simulink model "YawRateController"  (R2024b)
settings: Solver=VariableStepAuto  StartTime=0.0  StopTime=10.0  RelTol=1e-3
libraries: slpidlib x1, vehdynlibscenariocommon x1, autolibshared x1
settings Model: Creator=aditya  LastModifiedBy=aditya

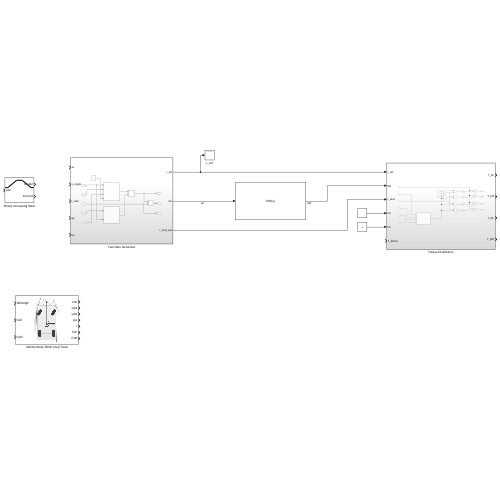
[thumbnail: Simulink's stored preview of the top-level diagram]
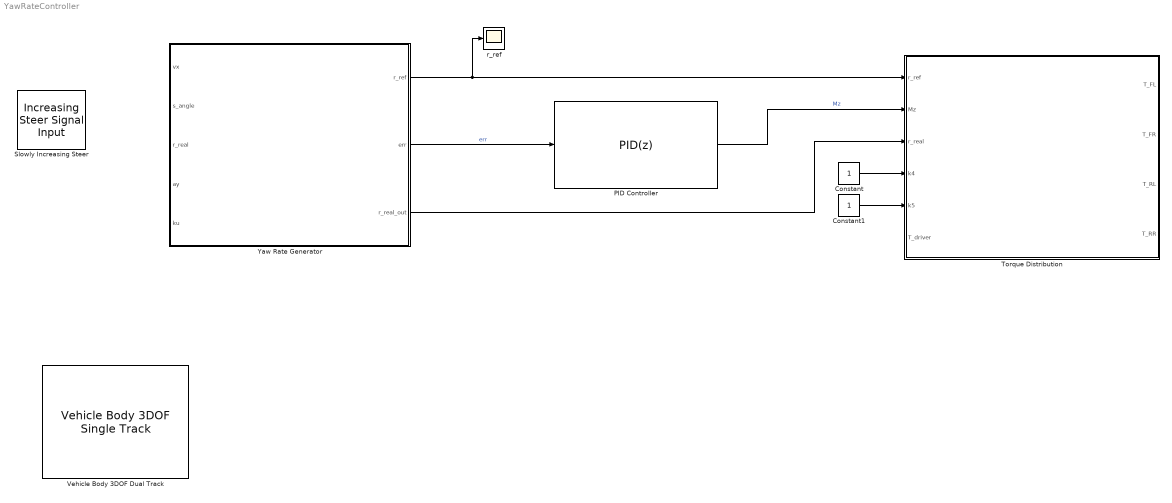
== system YawRateController ==
  Constant : Constant
  Constant1 : Constant
  PID Controller : slpidlib/PID Controller  Controller=PID  Form=Parallel  TimeDomain=Discrete-time  UseExternalTs=off  SampleTime=-1  IntegratorMethod=Forward Euler  FilterMethod=Forward Euler  ControllerParametersSource=internal  P=1  I=0  UseKiTs=off  D=0  UseExternalDerivativeSource=off  N=100  UseFilter=on  TunerSelectOption=Transfer Function Based (PID Tuner App)  InitialConditionSource=internal  InitialConditionForIntegrator=0  InitialConditionForFilter=0  DifferentiatorICPrevScaledInput=0  ExternalReset=none  TrackingMode=off  Kt=1  LimitOutput=off  SatLimitsSource=internal  UpperSaturationLimit=inf  LowerSaturationLimit=-inf  LinearizeAsGain=on  AntiWindupMode=none  Kb=1  LimitIntegrator=off  UpperIntegratorSaturationLimit=inf  LowerIntegratorSaturationLimit=-inf  POutMin=[]  POutMax=[]  IOutMin=[]  IOutMax=[]  DOutMin=[]  DOutMax=[]  NOutMin=[]  NOutMax=[]  SumOutMin=[]  SumOutMax=[]  SaturationOutMin=[]  SaturationOutMax=[]  PParamMin=[]  PParamMax=[]  IParamMin=[]  IParamMax=[]  DParamMin=[]  DParamMax=[]  NParamMin=[]  NParamMax=[]  KbParamMin=[]  KbParamMax=[]  KtParamMin=[]  KtParamMax=[]  KbOutMin=[]  KbOutMax=[]  KtOutMin=[]  KtOutMax=[]  IntegratorOutMin=[]  IntegratorOutMax=[]  FilterOutMin=[]  FilterOutMax=[]  SumI1OutMin=[]  SumI1OutMax=[]  SumI2OutMin=[]  SumI2OutMax=[]  SumI3OutMin=[]  SumI3OutMax=[]  SumI4OutMin=[]  SumI4OutMax=[]  SumDOutMin=[]  SumDOutMax=[]  DifferentiatorOutMin=[]  DifferentiatorOutMax=[]  FilterDiffOutCoefMin=[]  FilterDiffOutCoefMax=[]  ReciprocalOutMin=[]  ReciprocalOutMax=[]  SumDenOutMin=[]  SumDenOutMax=[]  SumNumOutMin=[]  SumNumOutMax=[]  DivideOutMin=[]  DivideOutMax=[]  UdiffTsProdOutMin=[]  UdiffTsProdOutMax=[]  NTsProdOutMin=[]  NTsProdOutMax=[]  UintegralTsProdOutMin=[]  UintegralTsProdOutMax=[]  UngainTsProdOutMin=[]  UngainTsProdOutMax=[]  ClampingZeroOutDataTypeStr=Inherit: Inherit via back propagation  ClampingZeroOutMin=[]  ClampingZeroOutMax=[]  FilterDenConstantOutDataTypeStr=Inherit: Inherit via back propagation  FilterDenConstantOutMin=[]  FilterDenConstantOutMax=[]  PCopyOutDataTypeStr=Inherit: Inherit via back propagation  PCopyOutMin=[]  PCopyOutMax=[]  NCopyOutDataTypeStr=Inherit: Inherit via back propagation  NCopyOutMin=[]  NCopyOutMax=[]  IntegratorContinuousStateAttributes=''  IntegratorStateMustResolveToSignalObject=off  IntegratorRTWStateStorageClass=Auto  FilterContinuousStateAttributes=''  FilterStateMustResolveToSignalObject=off  FilterRTWStateStorageClass=Auto  ParallelPVariant=InternalParameters  IdealPVariant=Disabled  IVariant=InternalParameters  DVariant=InternalParameters  IntegratorVariant=Discrete  SatVariant=Disabled  AWVariant=Passthrough  PCopyVariant=Disabled  TRVariant=Disabled  FdbkBlocksVariant=Forward  IdealPFdbkVariant=Disabled  SatFdbkVariant=Disabled  DerivativeFilterVariant=ForwardEulerFilter  NVariant=InternalParameters  NCopyVariant=Disabled  FilterICVariant=InternalICsFilter  IntegratorICVariant=InternalICs  ExternalResetVariant=Disabled  TRSumVariant=Passthrough  SumFdbkVariant=Disabled  SumVariant=Sum_PID  TsampFilterVariant=InternalTs  TsampNgainVariant=Passthrough  TsampIntegralVariant=Disabled_SignalSpec  ExternalSaturationOutDataTypeStr=Inherit: Same as second input  DerivativeSourceVariant=ErrorSignal  PreIntVariant=InternalPreInt
  Slowly Increasing Steer : vehdynlibscenariocommon/Increasing Steer Signal Input  ssMode=Initialize from model  ssVar=is50mph  tStart=2  velRef=50  velRefUnit=mph  steerRate=10  steerAmp=100  tDwellSteer=0  ayMax=.5  steerDir=Right  ayStop=off  ssDefault=on  X_o=0  Y_o=0  psi_o=0  ssTol=.1  ssMaxTime=30  ssWSName=is50mph  aMode=2
      settings: LibrarySourceBlock=vehdynlibscenario/Slowly Increasing Steer
  Torque Distribution : Subsystem
  Vehicle Body 3DOF Dual Track : autolibshared/Vehicle Body 3DOF Single Track  trackMode=Dual  inputMode=External forces  frontSteerMode=on  rearSteerMode=off  windMode=off  muMode=off  extFMode=off  extMMode=off  htchFMode=off  htchMMode=off  extXo=off  extpsio=off  extxdoto=off  extro=off  extYo=off  extTamb=off  extydoto=off  aMode=2  NF=2  NR=2  m=295  a=0.85  b=0.7  h=0.4  dh=1  hh=0.2  X_o=0  xdot_o=0  CalphaMode=off  sigmaMode=on  d=0  hl=0  w=[1.1,1.1]  Cy_f=12e3  Cy_r=11e3  sigma_f=.1  sigma_r=.1  alpha_f_brk=[-.1 .1]  Cy_f_data=[-9e3 9e3]  alpha_r_brk=[-.1 .1]  Cy_r_data=[-9e3 9e3]  Y_o=0  ydot_o=0  Izz=4000  psi_o=0  r_o=0  Af=0.728  Cd=0.85  Cl=.1  Cpm=.1  beta_w=[0 0.01:0.01:0.3]  Cs=[0:0.03:0.9]  Cym=[0 1e-6:0.01:0.3]  Pabs=101325  Tair=273  g=9.81  mu=1  xdot_tol=.01  Fznom=5000  Fxtire_sat=7e4  Fytire_sat=7e4  longOff=0  latOff=0  vertOff=0  wrapAng=off
      settings: LibrarySourceBlock=vehdynlibeom/Vehicle Body 3DOF Dual Track
  Yaw Rate Generator : Subsystem
  r_ref : Scope
  wires:
  Yaw Rate Generator/2(err) -> PID Controller/1  "err"
  PID Controller/1 -> Torque Distribution/2(Mz)  "Mz"
  Yaw Rate Generator/3(r_real_out) -> Torque Distribution/3(r_real)
  Yaw Rate Generator/1(r_ref) -> r_ref/1, Torque Distribution/1(r_ref)
  Constant/1 -> Torque Distribution/4(k4)
  Constant1/1 -> Torque Distribution/5(k5)

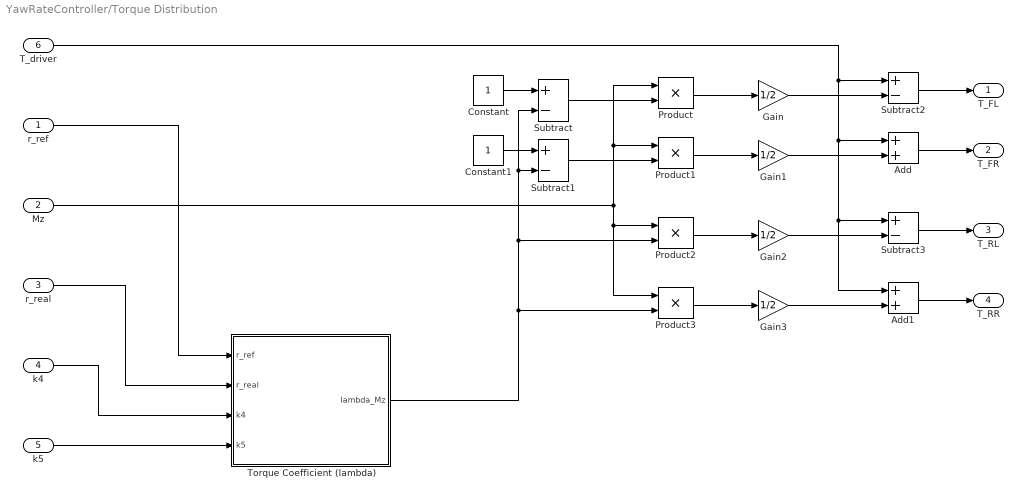
== system YawRateController/Torque Distribution ==
  r_ref : Inport
  Mz : Inport  Port=2
  r_real : Inport  Port=3
  k4 : Inport  Port=4
  k5 : Inport  Port=5
  T_driver : Inport  Port=6
  Add : Sum
  Add1 : Sum
  Constant : Constant
  Constant1 : Constant
  Gain{,1..3} (4 alike) : Gain  Gain=1/2
  Product{,1..3} (4 alike) : Product
  Subtract{,1..3} (4 alike) : Sum  Inputs=+-
  Torque Coefficient (lambda) : MATLAB Function  TreatAsAtomicUnit=on
  T_FL : Outport
  T_FR : Outport  Port=2
  T_RL : Outport  Port=3
  T_RR : Outport  Port=4
  wires:
  k4/1 -> Torque Coefficient (lambda)/3(k4)
  k5/1 -> Torque Coefficient (lambda)/4(k5)
  r_real/1 -> Torque Coefficient (lambda)/2(r_real)
  r_ref/1 -> Torque Coefficient (lambda)/1(r_ref)
  Constant1/1 -> Subtract1/1
  Subtract1/1 -> Product1/2
  Mz/1 -> Product2/1, Product3/1, Product1/1, Product/1
  Torque Coefficient (lambda)/1(lambda_Mz) -> Product3/2, Product2/2, Subtract/2, Subtract1/2
  Product1/1 -> Gain1/1
  Product2/1 -> Gain2/1
  Gain1/1 -> Add/2
  T_driver/1 -> Subtract2/1, Add/1, Add1/1, Subtract3/1
  Add1/1 -> T_RR/1
  Subtract3/1 -> T_RL/1
  Add/1 -> T_FR/1
  Subtract2/1 -> T_FL/1
  Constant/1 -> Subtract/1
  Subtract/1 -> Product/2
  Product/1 -> Gain/1
  Gain/1 -> Subtract2/2
  Product3/1 -> Gain3/1
  Gain3/1 -> Add1/2
  Gain2/1 -> Subtract3/2

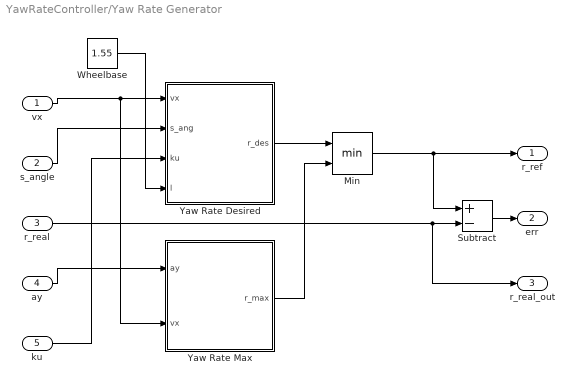
== system YawRateController/Yaw Rate Generator ==
  vx : Inport
  s_angle : Inport  Port=2
  r_real : Inport  Port=3
  ay : Inport  Port=4
  ku : Inport  Port=5
  Min : MinMax  Inputs=2
  Subtract : Sum  Inputs=+-
  Wheelbase : Constant  Value=1.55
  Yaw Rate Desired : MATLAB Function  TreatAsAtomicUnit=on
  Yaw Rate Max : MATLAB Function  TreatAsAtomicUnit=on
  r_ref : Outport
  err : Outport  Port=2
  r_real_out : Outport  Port=3
  wires:
  vx/1 -> Yaw Rate Desired/1(vx), Yaw Rate Max/2(vx)
  s_angle/1 -> Yaw Rate Desired/2(s_ang)
  Wheelbase/1 -> Yaw Rate Desired/4(l)
  ku/1 -> Yaw Rate Desired/3(ku)
  ay/1 -> Yaw Rate Max/1(ay)
  Yaw Rate Desired/1(r_des) -> Min/1
  Yaw Rate Max/1(r_max) -> Min/2
  Min/1 -> r_ref/1, Subtract/1
  r_real/1 -> Subtract/2, r_real_out/1
  Subtract/1 -> err/1

== matlab function YawRateController/Yaw Rate Generator/Yaw Rate Max ==
  data: ay input; r_max output; vx input
function r_max = yaw_rate_max(ay, vx)

r_max = abs(ay, vx);

== matlab function YawRateController/Yaw Rate Generator/Yaw Rate Desired ==
  data: vx input; r_des output; s_ang input; ku input; l input
function r_des = yaw_rate_des(vx, s_ang, ku, l)

r_des = (vx * s_ang) / (l + ku * (vx ^ 2));

== matlab function YawRateController/Torque Distribution/Torque Coefficient (lambda) ==
  data: r_ref input; r_real input; lambda_Mz output; k4 input; k5 input
function lambda_Mz = torque_lambda(r_ref, r_real, k4, k5)

lambda_Mz = (1 / (k5 - k4)) * (abs(r_ref) - abs(r_real) - k4);

if lambda_Mz <= k4
    lambda_Mz = 0;
elseif (lambda_Mz >= k5)
    lambda_Mz = 1;
end
